simulink model "Four_bit_Register"  (R2015a)
settings: Solver=ode45  StartTime=0.0  StopTime=2  RelTol=1e-3
libraries: simulink_extras x5
settings Model: Creator=citd  LastModifiedBy=citd

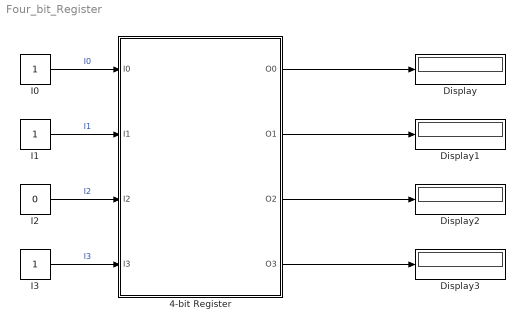
== system Four_bit_Register ==
  4-bit Register : Subsystem
  Display{,1..3} (4 alike) : Display
  I0 : Constant  OutDataTypeStr=boolean
  I1 : Constant  OutDataTypeStr=boolean
  I2 : Constant  Value=0  OutDataTypeStr=boolean
  I3 : Constant  OutDataTypeStr=boolean
  wires:
  I0/1 -> 4-bit Register/1(I0)  "I0"
  I1/1 -> 4-bit Register/2(I1)  "I1"
  I2/1 -> 4-bit Register/3(I2)  "I2"
  I3/1 -> 4-bit Register/4(I3)  "I3"
  4-bit Register/1(O0) -> Display/1
  4-bit Register/2(O1) -> Display1/1
  4-bit Register/3(O2) -> Display2/1
  4-bit Register/4(O3) -> Display3/1

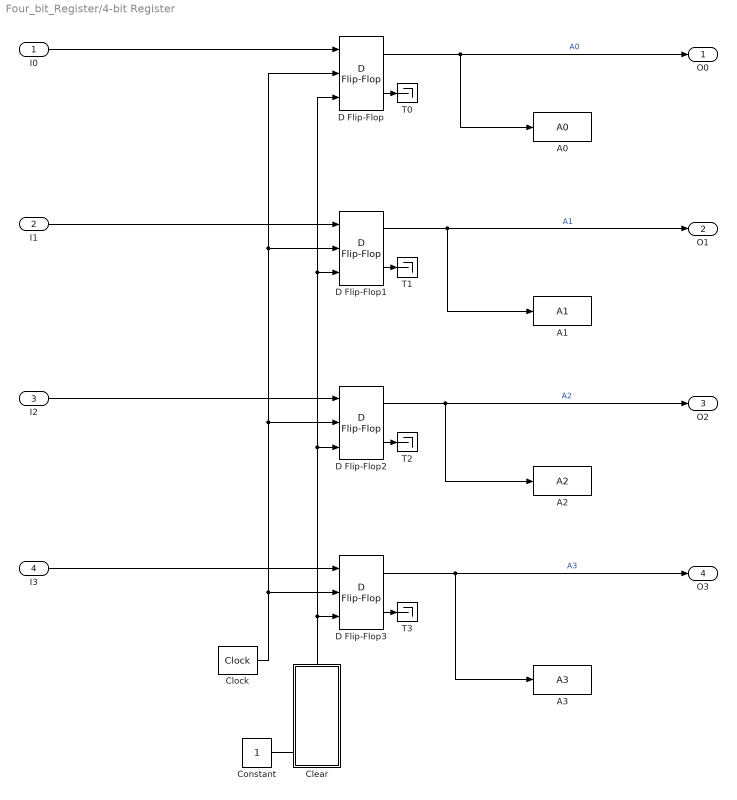
== system Four_bit_Register/4-bit Register ==
  I0 : Inport
  I1 : Inport  Port=2
  I2 : Inport  Port=3
  I3 : Inport  Port=4
  A0 : ToWorkspace  VariableName=A0  SampleTime=-1
      settings: MaxDataPoints=1  Save2DSignal=2-D array (concatenate along first dimension)
  A1 : ToWorkspace  VariableName=A1  SampleTime=-1
      settings: MaxDataPoints=1  Save2DSignal=2-D array (concatenate along first dimension)
  A2 : ToWorkspace  VariableName=A2  SampleTime=-1
      settings: MaxDataPoints=1  Save2DSignal=2-D array (concatenate along first dimension)
  A3 : ToWorkspace  VariableName=A3  SampleTime=-1
      settings: MaxDataPoints=1  Save2DSignal=2-D array (concatenate along first dimension)
  Clear : Subsystem  DialogController=hmiCreateDDGDialog  IsWebBlock=on  mask(MathWorksWebBlock){webBlockId=f428881a-90a5-4252-905e-1604b1fd28fe, webBlockType=toggleswitch, ShowInLibBrowser=on, ShowInitialText=on, HMISrcModelName=Four_bit_Register}
      mask prompts: webBlockId "WebBlock Id"; webBlockType "WebBlock Type"; HMISrcModelName "Source Model"
      mask Help: helpview([docroot '/mapfiles/simulink.map'], 'hmi_toggle_switch')
      mask Display:
      | if strcmp(get_param(bdroot(gcb),'BlockDiagramType'), 'library')
      |     image([(matlabroot) '/toolbox/simulink/hmi/icons/ToggleSwitch.png']);
      | end
  Clock : simulink_extras/Flip Flops/Clock  period=2
  Constant : Constant  OutDataTypeStr=boolean
  D Flip-Flop{,1..3} (4 alike) : simulink_extras/Flip Flops/D Flip-Flop
  T{0..3} (4 alike) : Terminator
  O0 : Outport
  O1 : Outport  Port=2
  O2 : Outport  Port=3
  O3 : Outport  Port=4
  wires:
  I1/1 -> D Flip-Flop1/1
  D Flip-Flop3/1 -> O3/1, A3/1  "A3"
  D Flip-Flop1/1 -> O1/1, A1/1  "A1"
  I2/1 -> D Flip-Flop2/1
  I0/1 -> D Flip-Flop/1
  I3/1 -> D Flip-Flop3/1
  D Flip-Flop/1 -> O0/1, A0/1  "A0"
  D Flip-Flop2/1 -> O2/1, A2/1  "A2"
  Clock/1 -> D Flip-Flop3/2, D Flip-Flop2/2, D Flip-Flop1/2, D Flip-Flop/2
  Constant/1 -> D Flip-Flop3/3, D Flip-Flop2/3, D Flip-Flop1/3, D Flip-Flop/3
  D Flip-Flop3/2 -> T3/1
  D Flip-Flop2/2 -> T2/1
  D Flip-Flop1/2 -> T1/1
  D Flip-Flop/2 -> T0/1

== system Four_bit_Register/4-bit Register/Clear ==
